simulink model "SMC"  (R2022b)
settings: Solver=FixedStepAuto  StartTime=0.0  StopTime=10.0  FixedStep=0.01  RelTol=1e-3
settings Model: Creator=Miakho  LastModifiedBy=Miakho
settings SolverCC: ZeroCrossAlgorithm=Adaptive
settings DebuggingCC: IgnoredZcDiagnostic=none

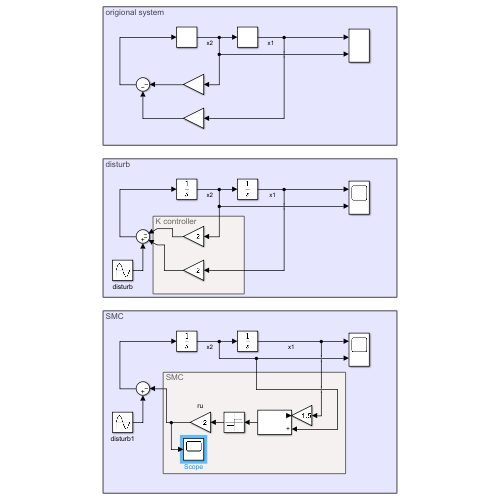
[thumbnail: Simulink's stored preview of the top-level diagram]
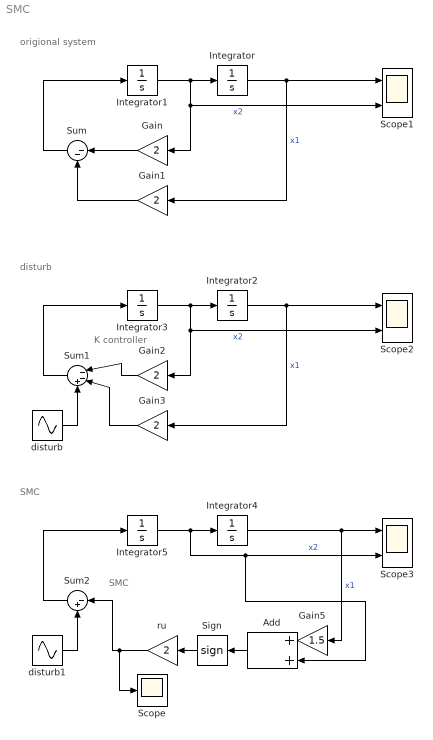
== system SMC ==
  note: SMC
  note: K controller
  note: origional system
  note: disturb
  note: SMC
  Add : Sum
  Gain{,1..3} (4 alike) : Gain  Gain=2
  Gain5 : Gain  Gain=1.5
  Integrator : Integrator  InitialCondition=1
  Integrator1 : Integrator  InitialCondition=-2
  Integrator2 : Integrator  InitialCondition=1
  Integrator3 : Integrator  InitialCondition=-2
  Integrator4 : Integrator  InitialCondition=1
  Integrator5 : Integrator  InitialCondition=-2
  Scope : Scope
  Scope1 : Scope  NumInputPorts=2
  Scope2 : Scope  NumInputPorts=2
  Scope3 : Scope  NumInputPorts=2
  Sign : Signum
  Sum : Sum  Inputs=|--
  Sum1 : Sum  Inputs=|--+
  Sum2 : Sum  Inputs=|-+
  disturb : Sin  Amplitude=0.2  SampleTime=0
  disturb1 : Sin  Amplitude=0.2  SampleTime=0
  ru : Gain  Gain=2
  wires:
  Integrator1/1 -> Gain/1, Scope1/2, Integrator/1  "x2"
  Integrator/1 -> Gain1/1, Scope1/1  "x1"
  Gain/1 -> Sum/1
  Gain1/1 -> Sum/2
  Sum/1 -> Integrator1/1
  Sum1/1 -> Integrator3/1
  Gain3/1 -> Sum1/2
  Gain2/1 -> Sum1/1
  Integrator2/1 -> Scope2/1, Gain3/1  "x1"
  Integrator3/1 -> Integrator2/1, Scope2/2, Gain2/1  "x2"
  disturb/1 -> Sum1/3
  disturb1/1 -> Sum2/2
  Integrator5/1 -> Add/2, Scope3/2, Integrator4/1  "x2"
  Integrator4/1 -> Gain5/1, Scope3/1  "x1"
  ru/1 -> Sum2/1, Scope/1
  Sum2/1 -> Integrator5/1
  Sign/1 -> ru/1
  Add/1 -> Sign/1
  Gain5/1 -> Add/1
